simulink model "Fm_complete"  (R2021a)
settings: Solver=VariableStepAuto  StartTime=0.0  StopTime=5  RelTol=1e-3
libraries: dsparch4 x1, commsynccomp2 x1
settings Model: Creator=mluser  LastModifiedBy=mluser
settings SolverCC: AlgebraicLoopSolver=TrustRegion
settings DebuggingCC: SFMachineParentedDataDiag=warning

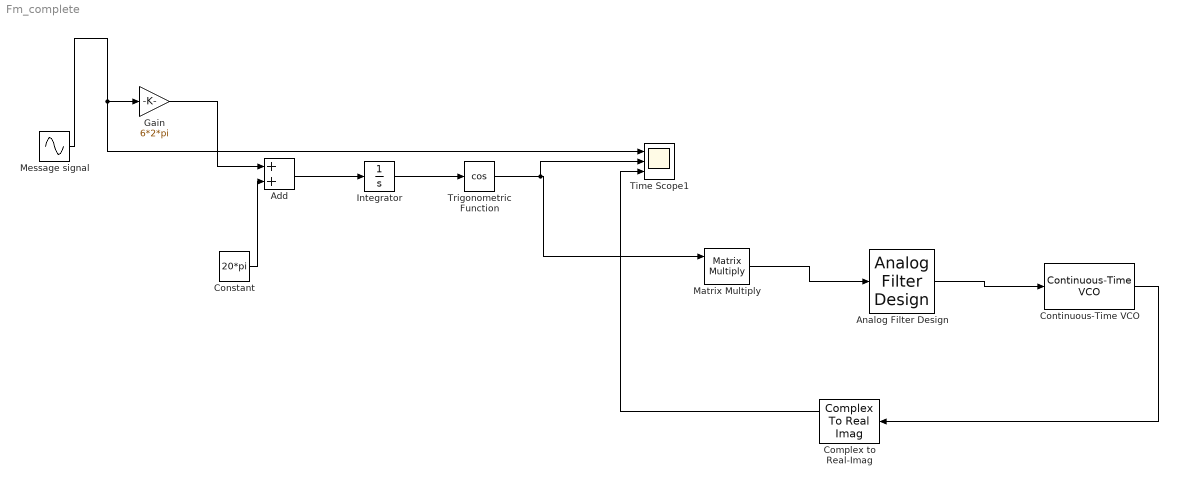
== system Fm_complete ==
  Add : Sum
  Analog Filter Design : dsparch4/Analog Filter Design  method=Butterworth  filttype=Lowpass  N=10  Wlo=2*pi*10  Whi=80  Rp=2  Rs=40
  Complex to Real-Imag : ComplexToRealImag
  Constant : Constant  Value=20*pi
  Continuous-Time VCO : commsynccomp2/Continuous-Time VCO  Ac=1  Fc=10  Kc=50  Ph=0
      settings: SourceProductBaseCode=CM
  Gain : Gain  Gain=6*2*pi
  Integrator : Integrator
  Matrix Multiply : Product  Multiplication=Matrix(*)
  Message signal : Sin  Frequency=20*pi  Phase=pi/2  SampleTime=1/5000
  Time Scope1 : Scope  NumInputPorts=3
  Trigonometric Function : Trigonometry  Operator=cos
  wires:
  Gain/1 -> Add/1
  Constant/1 -> Add/2
  Add/1 -> Integrator/1
  Integrator/1 -> Trigonometric Function/1
  Matrix Multiply/1 -> Analog Filter Design/1
  Analog Filter Design/1 -> Continuous-Time VCO/1
  Continuous-Time VCO/1 -> Complex to Real-Imag/1
  Message signal/1 -> Time Scope1/1, Gain/1
  Trigonometric Function/1 -> Time Scope1/2, Matrix Multiply/1
  Complex to Real-Imag/1 -> Time Scope1/3
